simulink model "LTI_aumentado"  (R2023a)
settings: Solver=VariableStepAuto  StartTime=0.0  StopTime=1  MaxStep=1e-4  RelTol=1e-3
undefined symbols (not defined in the file or in its folder): b_eq, Cts, J_eq, k_l, lambda, Ld, Lq, Pp, r, Rs_ref, Rts
libraries: SignalEditorBlockLib x3
settings Model: Creator=tobip  LastModifiedBy=tobip

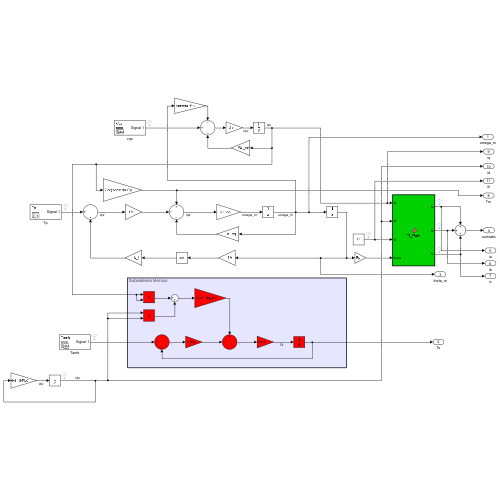
[thumbnail: Simulink's stored preview of the top-level diagram]
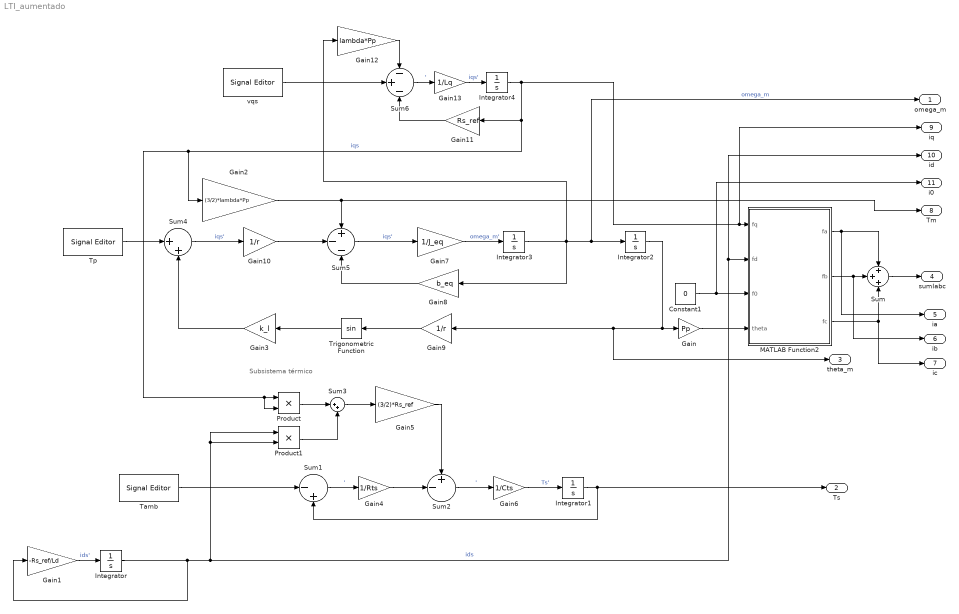
== system LTI_aumentado ==
  note: Subsistema térmico
  Constant1 : Constant  Value=0
  Gain : Gain  Gain=Pp
  Gain1 : Gain  Gain=-Rs_ref/Ld
  Gain10 : Gain  Gain=1/r
  Gain11 : Gain  Gain=Rs_ref
  Gain12 : Gain  Gain=lambda*Pp
  Gain13 : Gain  Gain=1/Lq
  Gain2 : Gain  Gain=(3/2)*lambda*Pp
  Gain3 : Gain  Gain=k_l
  Gain4 : Gain  Gain=1/Rts
  Gain5 : Gain  Gain=(3/2)*Rs_ref
  Gain6 : Gain  Gain=1/Cts
  Gain7 : Gain  Gain=1/J_eq
  Gain8 : Gain  Gain=b_eq
  Gain9 : Gain  Gain=1/r
  Integrator{,1..4} (5 alike) : Integrator
  MATLAB Function2 : MATLAB Function  TreatAsAtomicUnit=on
  Product : Product
  Product1 : Product
  Sum : Sum  Inputs=+++
  Sum1 : Sum  Inputs=|-+
  Sum2 : Sum  Inputs=+-|
  Sum3 : Sum  Inputs=|++
  Sum4 : Sum  Inputs=|++
  Sum5 : Sum  Inputs=+--
  Sum6 : Sum  Inputs=-+-
  Tamb : SignalEditorBlockLib/Signal Editor  FileName=senal_Tamb.mat  ActiveScenario=Tamb  ActiveSignal=Constant  IsBus=off  OutputBusObjectStr=Bus: BusObject  SampleTime=0  Interpolate=off  ZeroCross=off  OutputAfterFinalValue=Setting to zero  Unit=inherit  PreserveSignalName=on  ApplySigPropsToAllScenarios=on
  Tp : SignalEditorBlockLib/Signal Editor  FileName=senal_Tp.mat  ActiveScenario=Tp  ActiveSignal=Pulse  IsBus=off  OutputBusObjectStr=Bus: BusObject  SampleTime=0  Interpolate=off  ZeroCross=off  OutputAfterFinalValue=Setting to zero  Unit=inherit  PreserveSignalName=on  ApplySigPropsToAllScenarios=on
  Trigonometric Function : Trigonometry
  vqs : SignalEditorBlockLib/Signal Editor  FileName=senal_vqs.mat  ActiveScenario=Vqs  ActiveSignal=Pulse  IsBus=off  OutputBusObjectStr=Bus: BusObject  SampleTime=0  Interpolate=off  ZeroCross=off  OutputAfterFinalValue=Setting to zero  Unit=inherit  PreserveSignalName=on  ApplySigPropsToAllScenarios=on
  omega_m : Outport
  Ts : Outport  Port=2
  theta_m : Outport  Port=3
  sumIabc : Outport  Port=4
  ia : Outport  Port=5
  ib : Outport  Port=6
  ic : Outport  Port=7
  Tm : Outport  Port=8
  iq : Outport  Port=9
  id : Outport  Port=10
  i0 : Outport  Port=11
  wires:
  Integrator1/1 -> Ts/1, Sum1/2
  Integrator2/1 -> Gain/1, Gain9/1, theta_m/1
  Constant1/1 -> MATLAB Function2/3(f0), i0/1
  Gain/1 -> MATLAB Function2/4(theta)
  MATLAB Function2/1(fa) -> Sum/1, ia/1
  MATLAB Function2/2(fb) -> Sum/2, ib/1
  MATLAB Function2/3(fc) -> ic/1, Sum/3
  Sum/1 -> sumIabc/1
  Gain1/1 -> Integrator/1  "ids'"
  Integrator/1 -> Gain1/1, Product1/1, Product1/2, MATLAB Function2/2(fd), id/1  "ids"
  Gain2/1 -> Tm/1, Sum5/1
  Sum3/1 -> Gain5/1
  Product/1 -> Sum3/1
  Product1/1 -> Sum3/2
  Tamb/1 -> Sum1/1
  Sum1/1 -> Gain4/1  "'"
  Sum2/1 -> Gain6/1  "'"
  Gain6/1 -> Integrator1/1  "Ts'"
  Gain4/1 -> Sum2/2
  Gain5/1 -> Sum2/1
  Gain9/1 -> Trigonometric Function/1
  Gain10/1 -> Sum5/2
  Gain3/1 -> Sum4/2
  Sum5/1 -> Gain7/1  "iqs'"
  Trigonometric Function/1 -> Gain3/1
  Sum4/1 -> Gain10/1  "iqs'"
  Tp/1 -> Sum4/1
  Gain7/1 -> Integrator3/1  "omega_m'"
  Integrator3/1 -> Gain12/1, Integrator2/1, omega_m/1, Gain8/1  "omega_m"
  Gain8/1 -> Sum5/3
  Integrator4/1 -> Gain2/1, Product/2, Product/1, Gain11/1, iq/1, MATLAB Function2/1(fq)  "iqs"
  Gain12/1 -> Sum6/1
  vqs/1 -> Sum6/2
  Gain11/1 -> Sum6/3
  Sum6/1 -> Gain13/1  "'"
  Gain13/1 -> Integrator4/1  "iqs'"

== matlab function LTI_aumentado/MATLAB Function2 ==
  data: fq input; fa output size=1; fd input; f0 input; theta input; fb output size=1; fc output size=1
function [fa,fb,fc] = TI_Park(fq,fd,f0,theta)

f = [     cos(theta)              sin(theta)         1;
       cos(theta - (2*pi)/3)   sin(theta - (2*pi)/3)   1;
       cos(theta + (2*pi)/3)   sin(theta + (2*pi)/3)   1];

resultados = f*[fq;fd;f0];
fa = resultados(1);
fb = resultados(2);
fc = resultados(3);
